simulink library "attitude_library"  (R2021a)
settings: Solver=VariableStepAuto  StartTime=0.0  StopTime=10.0  RelTol=1e-3
libraries: $bdroot x9, vrlib x1
settings Model: Creator=Laura  LastModifiedBy=Laura

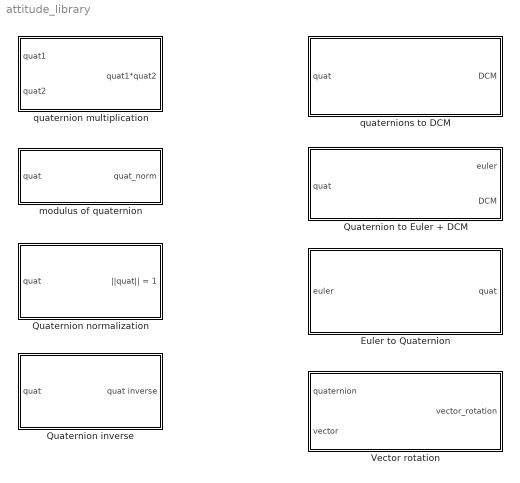
== system attitude_library ==
  Euler to Quaternion : Subsystem
  Quaternion inverse : Subsystem
  Quaternion normalization : Subsystem
  Quaternion to Euler + DCM : Subsystem
  Vector rotation : Subsystem
  modulus of quaternion : Subsystem
      settings: AttributesFormatString=modulus of quaternion
  quaternion multiplication : Subsystem
  quaternions to DCM : Subsystem

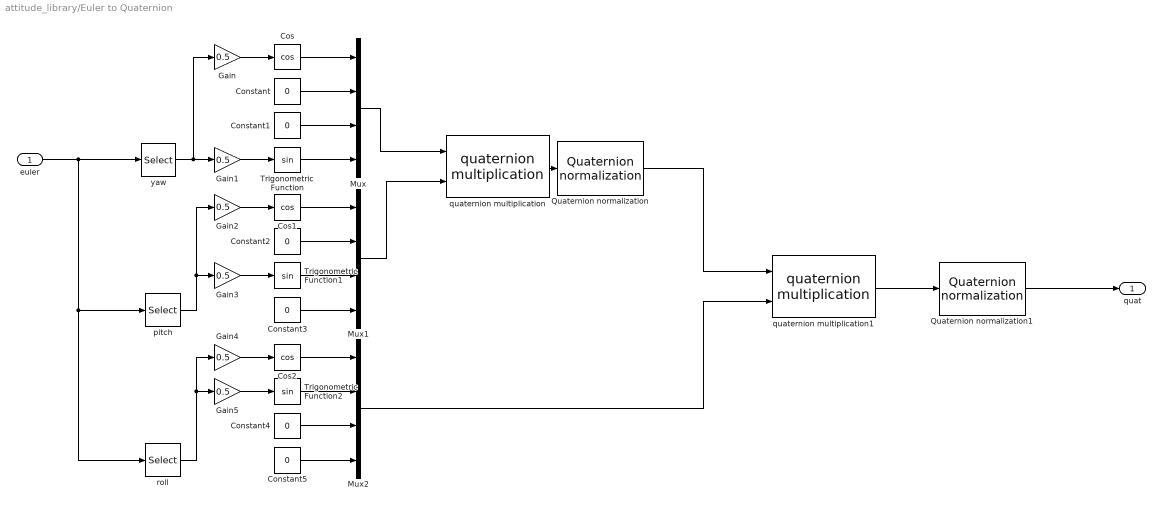
== system attitude_library/Euler to Quaternion ==
  euler : Inport
  Constant{,1..5} (6 alike) : Constant  Value=0
  Cos : Trigonometry  Operator=cos
  Cos1 : Trigonometry  Operator=cos
  Cos2 : Trigonometry  Operator=cos
  Gain{,1..5} (6 alike) : Gain  Gain=0.5
  Mux : Mux
  Mux1 : Mux
  Mux2 : Mux
  Quaternion normalization : $bdroot/Quaternion normalization  SystemSampleTime=-1  VariantActivationTime=update diagram  Latency=0  AutoFrameSizeCalculation=off
  Quaternion normalization1 : $bdroot/Quaternion normalization  SystemSampleTime=-1  VariantActivationTime=update diagram  Latency=0  AutoFrameSizeCalculation=off
  Trigonometric Function : Trigonometry
  Trigonometric Function1 : Trigonometry
  Trigonometric Function2 : Trigonometry
  pitch : Selector  InputPortWidth=3  IndexOptions=Index vector (dialog)  Indices=2  OutputSizes=1
  quaternion multiplication : $bdroot/quaternion multiplication  SystemSampleTime=-1  VariantActivationTime=update diagram  Latency=0  AutoFrameSizeCalculation=off
  quaternion multiplication1 : $bdroot/quaternion multiplication  SystemSampleTime=-1  VariantActivationTime=update diagram  Latency=0  AutoFrameSizeCalculation=off
  roll : Selector  InputPortWidth=3  IndexOptions=Index vector (dialog)  Indices=1  OutputSizes=1
  yaw : Selector  InputPortWidth=3  IndexOptions=Index vector (dialog)  Indices=3  OutputSizes=1
  quat : Outport
  wires:
  euler/1 -> roll/1, pitch/1, yaw/1
  yaw/1 -> Gain1/1, Gain/1
  Gain/1 -> Cos/1
  Gain1/1 -> Trigonometric Function/1
  Cos/1 -> Mux/1
  Constant/1 -> Mux/2
  Constant1/1 -> Mux/3
  Trigonometric Function/1 -> Mux/4
  pitch/1 -> Gain2/1, Gain3/1
  Cos1/1 -> Mux1/1
  Gain3/1 -> Trigonometric Function1/1
  Gain2/1 -> Cos1/1
  Constant2/1 -> Mux1/2
  roll/1 -> Gain4/1, Gain5/1
  Gain5/1 -> Trigonometric Function2/1
  Cos2/1 -> Mux2/1
  Gain4/1 -> Cos2/1
  Trigonometric Function2/1 -> Mux2/2
  Constant4/1 -> Mux2/3
  Constant5/1 -> Mux2/4
  Trigonometric Function1/1 -> Mux1/3
  Constant3/1 -> Mux1/4
  Mux/1 -> quaternion multiplication/1
  Mux1/1 -> quaternion multiplication/2
  Mux2/1 -> quaternion multiplication1/2
  quaternion multiplication/1 -> Quaternion normalization/1
  Quaternion normalization/1 -> quaternion multiplication1/1
  Quaternion normalization1/1 -> quat/1
  quaternion multiplication1/1 -> Quaternion normalization1/1

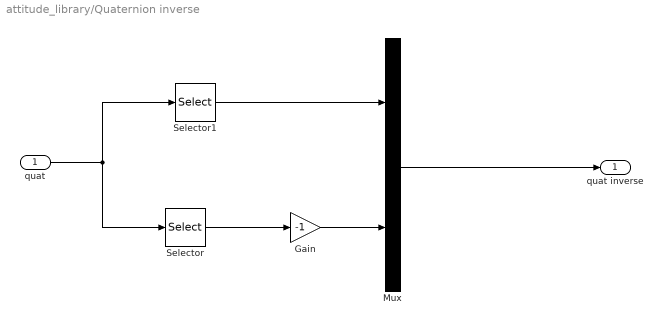
== system attitude_library/Quaternion inverse ==
  quat : Inport
  Gain : Gain  Gain=-1
  Mux : Mux  Inputs=2
  Selector : Selector  InputPortWidth=4  IndexOptions=Index vector (dialog)  Indices=[2 3 4]  OutputSizes=1
  Selector1 : Selector  InputPortWidth=4  IndexOptions=Index vector (dialog)  Indices=1  OutputSizes=1
  quat inverse : Outport
  wires:
  quat/1 -> Selector1/1, Selector/1
  Selector/1 -> Gain/1
  Mux/1 -> quat inverse/1
  Gain/1 -> Mux/2
  Selector1/1 -> Mux/1

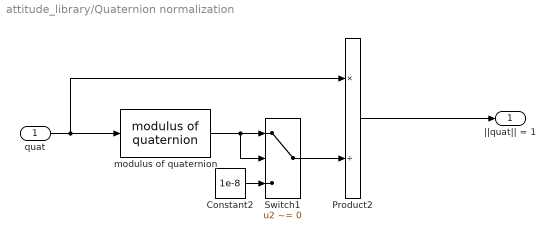
== system attitude_library/Quaternion normalization ==
  quat : Inport
  Constant2 : Constant  Value=1e-8  SampleTime=-1
  Product2 : Product  Inputs=*/  InputSameDT=on  RndMeth=Zero  SaturateOnIntegerOverflow=on  OutDataTypeStr=Inherit: Same as first input
  Switch1 : Switch  Criteria=u2 ~= 0
  modulus of quaternion : $bdroot/modulus of quaternion  SystemSampleTime=-1  VariantActivationTime=update diagram  Latency=0  AutoFrameSizeCalculation=off
      settings: AttributesFormatString=modulus of quaternion
  ||quat|| = 1 : Outport
  wires:
  quat/1 -> modulus of quaternion/1, Product2/1
  Constant2/1 -> Switch1/3
  Product2/1 -> ||quat|| = 1/1
  Switch1/1 -> Product2/2
  modulus of quaternion/1 -> Switch1/2, Switch1/1

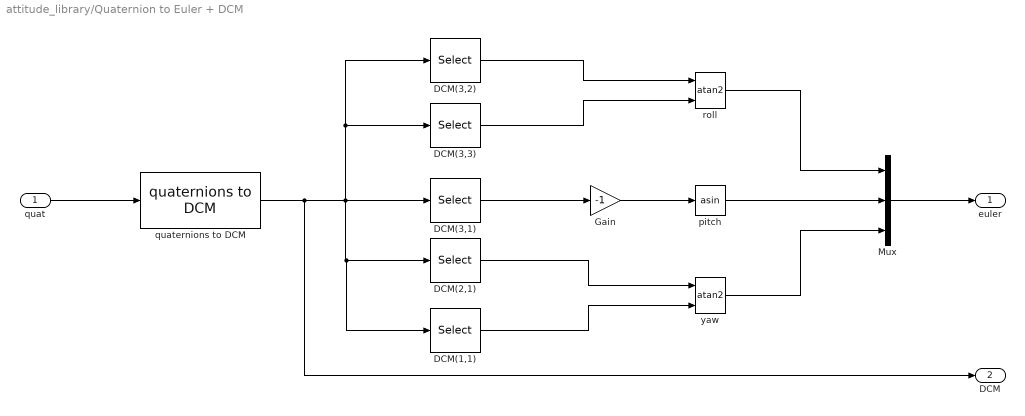
== system attitude_library/Quaternion to Euler + DCM ==
  quat : Inport
  DCM(1,1) : Selector  NumberOfDimensions=2  InputPortWidth=3  IndexOptions=Index vector (dialog),Index vector (dialog)  Indices=1,1  OutputSizes=1,1
  DCM(2,1) : Selector  NumberOfDimensions=2  InputPortWidth=3  IndexOptions=Index vector (dialog),Index vector (dialog)  Indices=2,1  OutputSizes=1,1
  DCM(3,1) : Selector  NumberOfDimensions=2  InputPortWidth=3  IndexOptions=Index vector (dialog),Index vector (dialog)  Indices=3,1  OutputSizes=1,1
  DCM(3,2) : Selector  NumberOfDimensions=2  InputPortWidth=3  IndexOptions=Index vector (dialog),Index vector (dialog)  Indices=3,2  OutputSizes=1,1
  DCM(3,3) : Selector  NumberOfDimensions=2  InputPortWidth=3  IndexOptions=Index vector (dialog),Index vector (dialog)  Indices=3,3  OutputSizes=1,1
  Gain : Gain  Gain=-1
  Mux : Mux  Inputs=3
  pitch : Trigonometry  Operator=asin
  quaternions to DCM : $bdroot/quaternions to DCM  SystemSampleTime=-1  VariantActivationTime=update diagram  Latency=0  AutoFrameSizeCalculation=off
  roll : Trigonometry  Operator=atan2
  yaw : Trigonometry  Operator=atan2
  euler : Outport
  DCM : Outport  Port=2
  wires:
  quaternions to DCM/1 -> DCM(3,2)/1, DCM(3,3)/1, DCM(3,1)/1, DCM(2,1)/1, DCM(1,1)/1, DCM/1
  quat/1 -> quaternions to DCM/1
  Mux/1 -> euler/1
  yaw/1 -> Mux/3
  pitch/1 -> Mux/2
  roll/1 -> Mux/1
  DCM(1,1)/1 -> yaw/2
  DCM(2,1)/1 -> yaw/1
  DCM(3,1)/1 -> Gain/1
  DCM(3,3)/1 -> roll/2
  DCM(3,2)/1 -> roll/1
  Gain/1 -> pitch/1

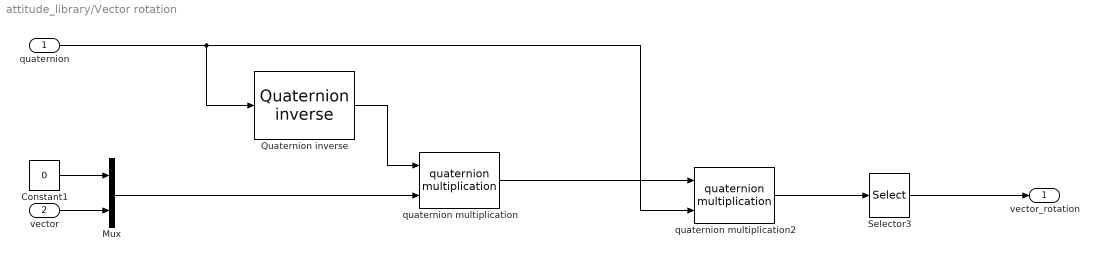
== system attitude_library/Vector rotation ==
  quaternion : Inport
  vector : Inport  Port=2
  Constant1 : Constant  Value=0
  Mux : Mux  Inputs=2
  Quaternion inverse : $bdroot/Quaternion inverse  SystemSampleTime=-1  VariantActivationTime=update diagram  Latency=0  AutoFrameSizeCalculation=off
  Selector3 : Selector  InputPortWidth=4  IndexOptions=Index vector (dialog)  Indices=[2 3 4]  OutputSizes=1
  quaternion multiplication : $bdroot/quaternion multiplication  SystemSampleTime=-1  VariantActivationTime=update diagram  Latency=0  AutoFrameSizeCalculation=off
  quaternion multiplication2 : $bdroot/quaternion multiplication  SystemSampleTime=-1  VariantActivationTime=update diagram  Latency=0  AutoFrameSizeCalculation=off
  vector_rotation : Outport
  wires:
  quaternion multiplication2/1 -> Selector3/1
  Mux/1 -> quaternion multiplication/2
  quaternion multiplication/1 -> quaternion multiplication2/1
  quaternion/1 -> Quaternion inverse/1, quaternion multiplication2/2
  Selector3/1 -> vector_rotation/1
  Constant1/1 -> Mux/1
  Quaternion inverse/1 -> quaternion multiplication/1
  vector/1 -> Mux/2

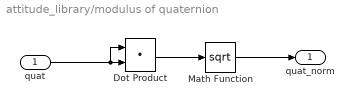
== system attitude_library/modulus of quaternion ==
  quat : Inport
  Dot Product : DotProduct  InputSameDT=on  OutDataTypeStr=Inherit: Inherit via internal rule
  Math Function : Math  Operator=sqrt  SignedPower=on  SaturateOnIntegerOverflow=on
  quat_norm : Outport  VectorParamsAs1DForOutWhenUnconnected=off
  wires:
  Dot Product/1 -> Math Function/1
  Math Function/1 -> quat_norm/1
  quat/1 -> Dot Product/1, Dot Product/2

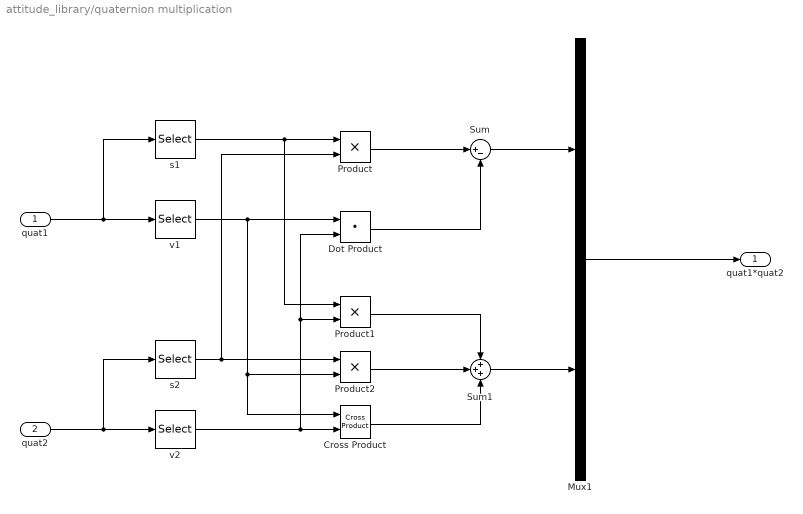
== system attitude_library/quaternion multiplication ==
  quat1 : Inport
  quat2 : Inport  Port=2
  Cross Product : vrlib/Utilities/Cross Product
  Dot Product : DotProduct  InputSameDT=on  OutDataTypeStr=Inherit: Inherit via internal rule
  Mux1 : Mux  Inputs=2
  Product : Product
  Product1 : Product
  Product2 : Product
  Sum : Sum  Inputs=|+-
  Sum1 : Sum  Inputs=+++
  s1 : Selector  InputPortWidth=4  IndexOptions=Index vector (dialog)  Indices=1  OutputSizes=1
  s2 : Selector  InputPortWidth=4  IndexOptions=Index vector (dialog)  Indices=1  OutputSizes=1
  v1 : Selector  InputPortWidth=4  IndexOptions=Index vector (dialog)  Indices=[2 3 4]  OutputSizes=1
  v2 : Selector  InputPortWidth=4  IndexOptions=Index vector (dialog)  Indices=[2 3 4]  OutputSizes=1
  quat1*quat2 : Outport
  wires:
  Mux1/1 -> quat1*quat2/1
  v2/1 -> Dot Product/2, Product1/2, Cross Product/2
  quat1/1 -> s1/1, v1/1
  quat2/1 -> v2/1, s2/1
  Cross Product/1 -> Sum1/3
  Product1/1 -> Sum1/1
  Sum/1 -> Mux1/1
  Product2/1 -> Sum1/2
  Sum1/1 -> Mux1/2
  Product/1 -> Sum/1
  s1/1 -> Product1/1, Product/1
  Dot Product/1 -> Sum/2
  s2/1 -> Product/2, Product2/1
  v1/1 -> Dot Product/1, Product2/2, Cross Product/1

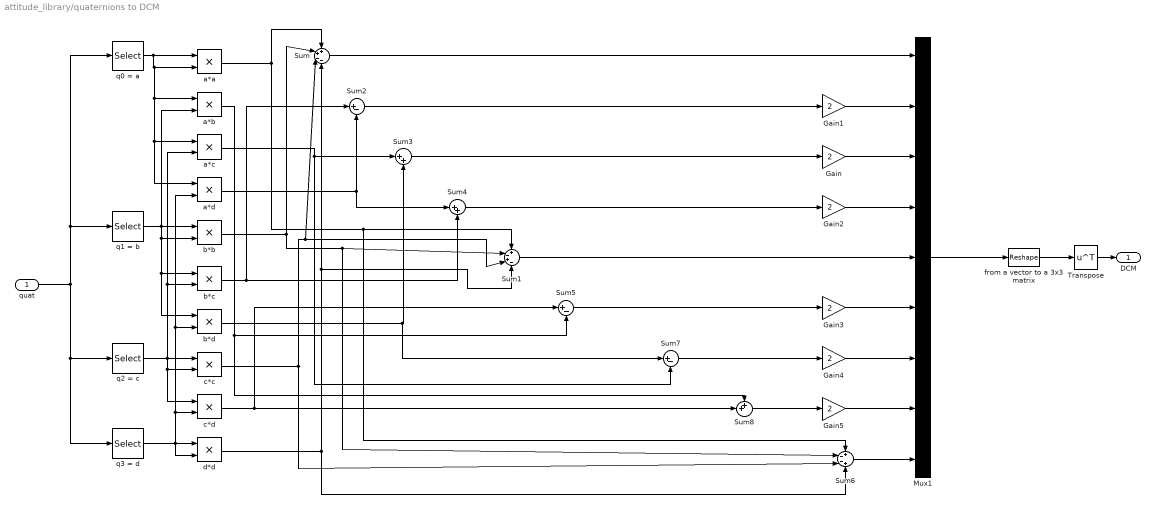
== system attitude_library/quaternions to DCM ==
  quat : Inport
  Gain{,1..5} (6 alike) : Gain  Gain=2
  Mux1 : Mux  Inputs=9
  Sum : Sum  Inputs=++--
  Sum1 : Sum  Inputs=+-+-
  Sum2 : Sum  Inputs=|+-
  Sum3 : Sum  Inputs=|++
  Sum4 : Sum  Inputs=|++
  Sum5 : Sum  Inputs=|+-
  Sum6 : Sum  Inputs=+--+
  Sum7 : Sum  Inputs=|+-
  Sum8 : Sum  Inputs=++|
  Transpose : Math  Operator=transpose  SaturateOnIntegerOverflow=on
  a*a : Product
  a*b : Product
  a*c : Product
  a*d : Product
  b*b : Product
  b*c : Product
  b*d : Product
  c*c : Product
  c*d : Product
  d*d : Product
  from a vector to a 3x3 matrix : Reshape  OutputDimensionality=Customize  OutputDimensions=[3,3]
  q0 = a : Selector  InputPortWidth=4  IndexOptions=Index vector (dialog)  Indices=1  OutputSizes=1
  q1 = b : Selector  InputPortWidth=4  IndexOptions=Index vector (dialog)  Indices=2  OutputSizes=1
  q2 = c : Selector  InputPortWidth=4  IndexOptions=Index vector (dialog)  Indices=3  OutputSizes=1
  q3 = d : Selector  InputPortWidth=4  IndexOptions=Index vector (dialog)  Indices=4  OutputSizes=1
  DCM : Outport
  wires:
  quat/1 -> q3 = d/1, q2 = c/1, q1 = b/1, q0 = a/1
  q0 = a/1 -> a*a/1, a*b/1, a*d/1, a*c/1, a*a/2
  q1 = b/1 -> b*d/1, b*c/1, b*b/2, a*b/2, b*b/1
  q2 = c/1 -> a*c/2, b*c/2, c*c/1, c*d/1, c*c/2
  q3 = d/1 -> b*d/2, a*d/2, c*d/2, d*d/1, d*d/2
  b*b/1 -> Sum1/2, Sum6/2, Sum/2
  Sum/1 -> Mux1/1
  c*c/1 -> Sum6/3, Sum1/3, Sum/3
  d*d/1 -> Sum6/4, Sum/4, Sum1/4
  a*a/1 -> Sum1/1, Sum6/1, Sum/1
  Sum1/1 -> Mux1/5
  Sum2/1 -> Gain1/1
  b*c/1 -> Sum4/2, Sum2/1
  a*d/1 -> Sum2/2, Sum4/1
  Sum3/1 -> Gain/1
  Sum4/1 -> Gain2/1
  Gain/1 -> Mux1/3
  Gain1/1 -> Mux1/2
  Gain2/1 -> Mux1/4
  a*c/1 -> Sum7/2, Sum3/1
  b*d/1 -> Sum7/1, Sum3/2
  Sum5/1 -> Gain3/1
  Gain3/1 -> Mux1/6
  c*d/1 -> Sum8/2, Sum5/1
  a*b/1 -> Sum5/2, Sum8/1
  Sum7/1 -> Gain4/1
  Gain4/1 -> Mux1/7
  Sum6/1 -> Mux1/9
  Gain5/1 -> Mux1/8
  Sum8/1 -> Gain5/1
  Mux1/1 -> from a vector to a 3x3 matrix/1
  from a vector to a 3x3 matrix/1 -> Transpose/1
  Transpose/1 -> DCM/1
